simulink model "example_design_enabled"  (R2017b)
settings: Solver=VariableStepAuto  StartTime=0.0  StopTime=10.0  RelTol=1e-3
libraries: simulink x2
settings Model: Creator=cyarp  LastModifiedBy=cyarp

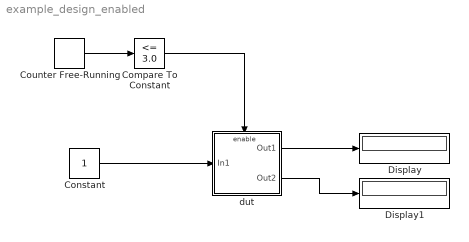
== system example_design_enabled ==
  Compare To Constant : simulink/Logic and Bit Operations/Compare To Constant  relop=<=  const=3.0  OutDataTypeStr=boolean
  Constant : Constant
  Counter Free-Running : simulink/Sources/Counter Free-Running  NumBits=16  tsamp=-1
  Display : Display
  Display1 : Display
  dut : Subsystem
  wires:
  Constant/1 -> dut/1(In1)
  dut/1(Out1) -> Display/1
  dut/2(Out2) -> Display1/1
  Counter Free-Running/1 -> Compare To Constant/1
  Compare To Constant/1 -> dut/Enable

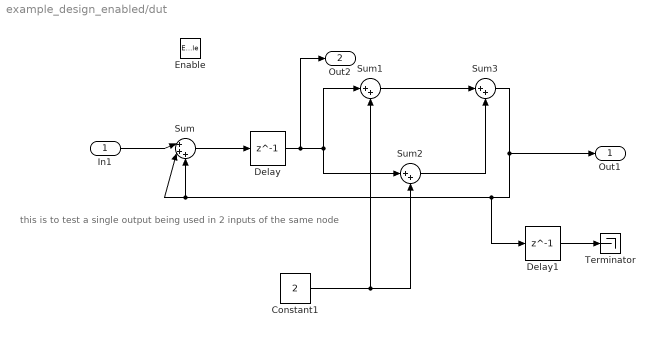
== system example_design_enabled/dut ==
  note: this is to test a single output being used in 2 inputs of the same node
  In1 : Inport
  Enable : EnablePort
  Constant1 : Constant  Value=2
  Delay : Delay  DelayLength=1  InitialCondition=0
  Delay1 : Delay  DelayLength=1  InitialCondition=0
  Sum : Sum  Inputs=|+++
  Sum1 : Sum  Inputs=|++
  Sum2 : Sum  Inputs=|++
  Sum3 : Sum  Inputs=|++
  Terminator : Terminator
  Out1 : Outport
  Out2 : Outport  Port=2
  wires:
  Sum/1 -> Delay/1
  In1/1 -> Sum/1
  Constant1/1 -> Sum2/2, Sum1/2
  Delay/1 -> Out2/1, Sum2/1, Sum1/1
  Sum1/1 -> Sum3/1
  Sum3/1 -> Out1/1, Delay1/1, Sum/3, Sum/2
  Sum2/1 -> Sum3/2
  Delay1/1 -> Terminator/1
